simulink model "Tiny_M6"  (R2017b)
settings: Solver=VariableStepAuto  StartTime=0.0  StopTime=10.0  RelTol=1e-3

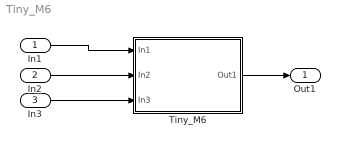
== system Tiny_M6 ==
  In1 : Inport
  In2 : Inport  Port=2
  In3 : Inport  Port=3
  Tiny_M6 : Subsystem
  Out1 : Outport
  wires:
  Tiny_M6/1(Out1) -> Out1/1
  In1/1 -> Tiny_M6/1(In1)
  In2/1 -> Tiny_M6/2(In2)
  In3/1 -> Tiny_M6/3(In3)

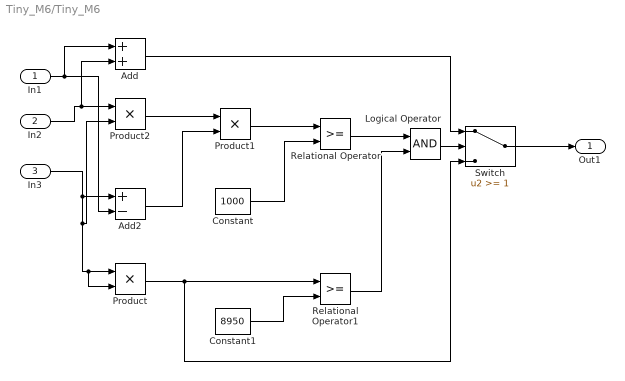
== system Tiny_M6/Tiny_M6 ==
  In1 : Inport
  In2 : Inport  Port=2
  In3 : Inport  Port=3
  Add : Sum
  Add2 : Sum  Inputs=+-
  Constant : Constant  Value=1000
  Constant1 : Constant  Value=8950
  Logical Operator : Logic  AllPortsSameDT=off  OutDataTypeStr=boolean
  Product : Product
  Product1 : Product
  Product2 : Product
  Relational Operator : RelationalOperator  OutDataTypeStr=boolean  RndMeth=Nearest
  Relational Operator1 : RelationalOperator  OutDataTypeStr=boolean  RndMeth=Nearest
  Switch : Switch  Threshold=1
  Out1 : Outport
  wires:
  In3/1 -> Add2/1, Product/2, Product/1, Product2/2
  In1/1 -> Add/1, Add2/2
  In2/1 -> Add/2, Product2/1
  Product2/1 -> Product1/1
  Add2/1 -> Product1/2
  Product1/1 -> Relational Operator/1
  Product/1 -> Switch/3, Relational Operator1/1
  Constant/1 -> Relational Operator/2
  Constant1/1 -> Relational Operator1/2
  Relational Operator/1 -> Logical Operator/1
  Relational Operator1/1 -> Logical Operator/2
  Logical Operator/1 -> Switch/2
  Add/1 -> Switch/1
  Switch/1 -> Out1/1
